simulink model "CONTROL_STARTER_2020b"  (R2020b)
settings: Solver=VariableStepAuto  StartTime=0.0  StopTime=10.0  RelTol=1e-3
settings Model: Creator=EGI-Z400  LastModifiedBy=HWRL user
settings DebuggingCC: SFMachineParentedDataDiag=error

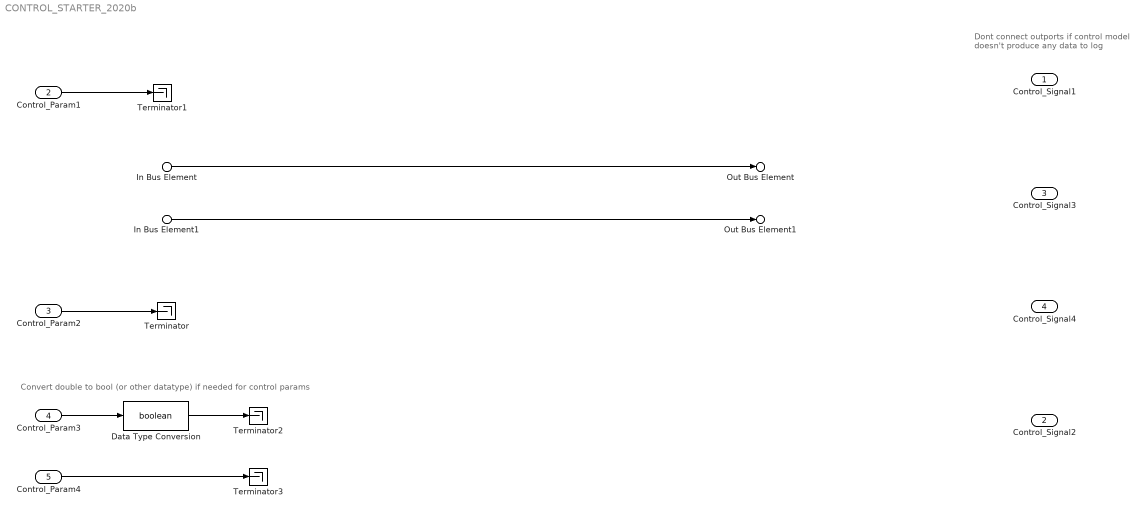
== system CONTROL_STARTER_2020b ==
  note: Convert double to bool (or other datatype) if needed for control params
  note: Dont connect outports if control
      | model doesn't produce any data
      | to log
  In Bus Element : Inport  PortName=twin2ctrl  Element=Pos_Aft
  In Bus Element1 : Inport  PortName=twin2ctrl  Element=Pos_Bow
  Control_Param1 : Inport  Port=2
  Control_Param2 : Inport  Port=3
  Control_Param3 : Inport  Port=4  OutDataTypeStr=double
  Control_Param4 : Inport  Port=5  OutDataTypeStr=double
  Data Type Conversion : DataTypeConversion  OutDataTypeStr=boolean
  Terminator{,1..3} (4 alike) : Terminator
  Control_Signal1 : Outport
  Control_Signal2 : Outport  Port=2
  Control_Signal3 : Outport  Port=3
  Control_Signal4 : Outport  Port=4
  Out Bus Element : Outport  Port=5  PortName=ctrl2twin  Element=Cur_Aft
  Out Bus Element1 : Outport  Port=5  PortName=ctrl2twin  Element=Cur_Bow
  wires:
  Control_Param3/1 -> Data Type Conversion/1
  Control_Param4/1 -> Terminator3/1
  In Bus Element1/1 -> Out Bus Element1/1
  In Bus Element/1 -> Out Bus Element/1
  Control_Param2/1 -> Terminator/1
  Control_Param1/1 -> Terminator1/1
  Data Type Conversion/1 -> Terminator2/1
